simulink model "Computer"  (Simulink 8.1)
settings: Solver=ode45  StartTime=0.0  StopTime=21  RelTol=1e-3
libraries: Common_Library x33, commutil2 x5, Computer_Library x3, simulink_extras x3
settings Model: Creator=N  LastModifiedBy=uzivatel
settings DataIOCC: LimitDataPoints=off  SignalLoggingSaveFormat=Dataset
settings OptimizationCC: ExpressionDepthLimit=128
settings DebuggingCC: UnderspecifiedInitializationDetection=Simplified  MergeDetectMultiDrivingBlocksExec=error  SolverPrmCheckMsg=none  FcnCallInpInsideContextMsg=EnableAllAsError  FrameProcessingCompatibilityMsg=error  StateNameClashWarn=none
settings HardwareCC: ProdBitPerPointer=64  ProdLargestAtomicFloat=Float  ProdIntDivRoundTo=Zero  ProdEndianess=LittleEndian  ProdHWDeviceType=Intel->x86-64 (Windows64)
settings ModelReferenceCC: PropagateSignalLabelsOutOfModel=on
settings GRTTargetCC: CodeReplacementLibrary=None  CombineOutputUpdateFcns=on  CPPClassGenCompliant=on  GRTInterface=off

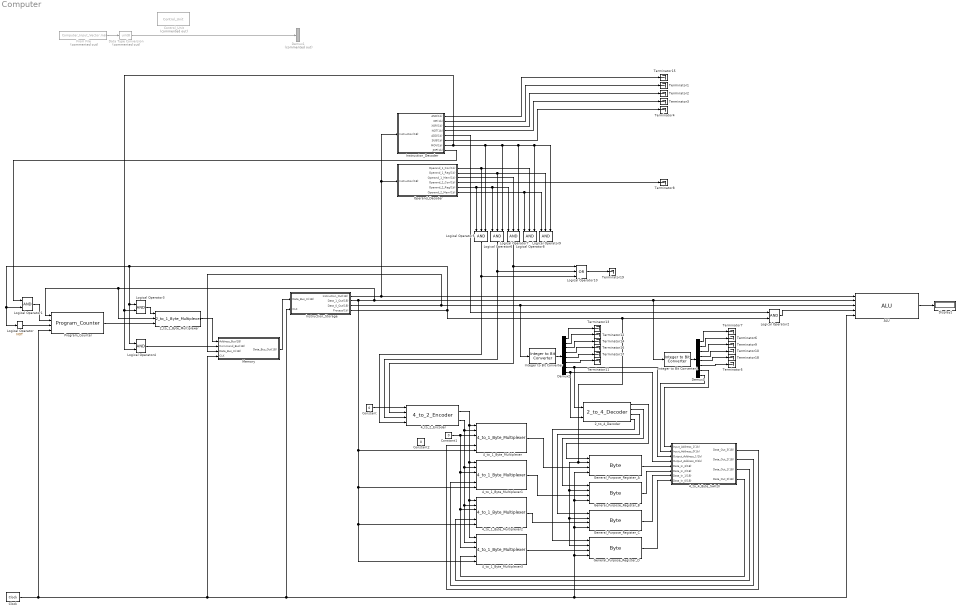
== system Computer ==
  2_to_1_Byte_Multiplexer : Common_Library/Multiplexers/2_to_1_Byte_Multiplexer
  2_to_4_Decoder : Common_Library/Decoders/2_to_4_Decoder
  4_to_1_Byte_Multiplexer{,1..3} (4 alike) : Common_Library/Multiplexers/4_to_1_Byte_Multiplexer
  4_to_2_Encoder : Common_Library/Encoders/4_to_2_Encoder
  4_to_4_Byte_Switch : Subsystem
  ALU : Computer_Library/ALU
  Clock : simulink_extras/Flip Flops/Clock  period=1
  Constant : Constant  Value=0  OutDataTypeStr=boolean
  Constant1 : Constant  Value=0  OutDataTypeStr=uint8
  Constant2 : Constant  Value=0  OutDataTypeStr=uint8
  Control_Unit : Computer_Library/Control_Unit  Commented=on
  Data Type Conversion : DataTypeConversion  Commented=on  OutDataTypeStr=uint8
  Demux1 : Demux  Commented=on  Outputs=2
  Demux2 : Demux  Outputs=8
  Demux3 : Demux  Outputs=8
  Display1 : Display
  From File : FromFile  Commented=on  FileName=Computer_Input_Vector.mat  OutDataTypeStr=double  SampleTime=1  ExtrapolationBeforeFirstDataPoint=Hold first value  ExtrapolationAfterLastDataPoint=Ground value
  General_Purpose_Register_A : Common_Library/Memory_Blocks/Byte
  General_Purpose_Register_B : Common_Library/Memory_Blocks/Byte
  General_Purpose_Register_C : Common_Library/Memory_Blocks/Byte
  General_Purpose_Register_D : Common_Library/Memory_Blocks/Byte
  Instruction_Decoder : Subsystem
  Instruction_Storage : Subsystem
  Integer to Bit Converter : commutil2/Integer to Bit Converter  nbits=8  signedInputValues=Unsigned  bitOrder=MSB first  outDtype=boolean
  Integer to Bit Converter1 : commutil2/Integer to Bit Converter  nbits=8  signedInputValues=Unsigned  bitOrder=MSB first  outDtype=boolean
  Logical Operator : Logic  Operator=NOT  IconShape=distinctive  AllPortsSameDT=off  OutDataTypeStr=boolean
  Logical Operator{1..4} (4 alike) : Logic  IconShape=distinctive  AllPortsSameDT=off  OutDataTypeStr=boolean
  Logical Operator10 : Logic  Operator=OR  Inputs=3  IconShape=distinctive  AllPortsSameDT=off  OutDataTypeStr=boolean
  Logical Operator{5..9} (5 alike) : Logic  Inputs=3  IconShape=distinctive  AllPortsSameDT=off  OutDataTypeStr=boolean
  Memory : Subsystem
  Operand_Decoder : Subsystem
  Program_Counter : Computer_Library/Program_Counter
  Terminator{1..19} (19 alike) : Terminator
  wires:
  Instruction_Storage/4(Process(1b)) -> Logical Operator4/1, Logical Operator3/1, Logical Operator/1, Logical Operator1/2, Logical Operator2/2, General_Purpose_Register_B/2, General_Purpose_Register_C/2, General_Purpose_Register_D/2, General_Purpose_Register_A/2
  Program_Counter/1 -> 2_to_1_Byte_Multiplexer/3
  Instruction_Storage/3(Data_0_Out(1B)) -> ALU/3, Integer to Bit Converter/1, Memory/3(Data_Bus_In(1B))
  Instruction_Decoder/8(JMP(1b)) -> Logical Operator1/1
  Instruction_Storage/2(Data_1_Out(1B)) -> 2_to_1_Byte_Multiplexer/2, Program_Counter/1, Integer to Bit Converter1/1, ALU/2, 4_to_1_Byte_Multiplexer3/6, 4_to_1_Byte_Multiplexer2/6, 4_to_1_Byte_Multiplexer1/6, 4_to_1_Byte_Multiplexer/6
  Memory/1(Data_Bus_Out(1B)) -> Instruction_Storage/1(Data_Bus_In(1B))
  Clock/1 -> Program_Counter/4, Memory/4(CLK), Instruction_Storage/2(CLK), ALU/5, General_Purpose_Register_A/4, General_Purpose_Register_B/4, General_Purpose_Register_C/4, General_Purpose_Register_D/4
  From File/1 -> Data Type Conversion/1
  Data Type Conversion/1 -> Demux1/1
  Instruction_Decoder/7(MOV(1b)) -> Logical Operator5/3, Logical Operator6/3, Logical Operator7/3, Logical Operator8/3, Logical Operator9/3, Logical Operator4/2, Logical Operator3/2
  Instruction_Storage/1(Instruction_Out(1B)) -> Operand_Decoder/1(Instruction(1B)), Instruction_Decoder/1(Instruction(1B)), ALU/1
  Logical Operator/1 -> Program_Counter/3
  Instruction_Decoder/5(ADD(1b)) -> Logical Operator2/1
  Logical Operator1/1 -> Program_Counter/2
  Logical Operator2/1 -> ALU/4
  2_to_1_Byte_Multiplexer/1 -> Memory/1(Address_Bus(1B))
  ALU/1 -> Display1/1
  Logical Operator3/1 -> 2_to_1_Byte_Multiplexer/1
  Logical Operator4/1 -> Memory/2(Command_Bus(1B))
  Instruction_Decoder/1(AND(1b)) -> Terminator15/1
  Instruction_Decoder/2(OR(1b)) -> Terminator1/1
  Instruction_Decoder/3(XOR(1b)) -> Terminator2/1
  Instruction_Decoder/4(NOT(1b)) -> Terminator3/1
  Instruction_Decoder/6(SUB(1b)) -> Terminator4/1
  Operand_Decoder/1(Operand_1_Con(1b)) -> Logical Operator8/2, Logical Operator5/2
  Operand_Decoder/2(Operand_1_Reg(1b)) -> Logical Operator6/2, Logical Operator9/2
  Operand_Decoder/3(Operand_1_Mem(1b)) -> Logical Operator7/2
  Operand_Decoder/4(Operand_2_Con(1b)) -> Terminator8/1
  Operand_Decoder/6(Operand_2_Mem(1b)) -> Logical Operator9/1, Logical Operator8/1
  2_to_4_Decoder/4 -> General_Purpose_Register_D/1
  2_to_4_Decoder/3 -> General_Purpose_Register_C/1
  2_to_4_Decoder/2 -> General_Purpose_Register_B/1
  2_to_4_Decoder/1 -> General_Purpose_Register_A/1
  Integer to Bit Converter/1 -> Demux2/1
  Demux2/8 -> 2_to_4_Decoder/2, 4_to_4_Byte_Switch/4(Output_Address_0(1b))
  Demux2/7 -> 2_to_4_Decoder/1, 4_to_4_Byte_Switch/3(Output_Address_1(1b))
  Demux2/1 -> Terminator13/1
  Demux2/2 -> Terminator12/1
  Demux2/3 -> Terminator14/1
  Demux2/4 -> Terminator16/1
  Demux2/5 -> Terminator17/1
  Demux2/6 -> Terminator11/1
  Operand_Decoder/5(Operand_2_Reg(1b)) -> Logical Operator7/1, Logical Operator6/1, Logical Operator5/1
  General_Purpose_Register_A/1 -> 4_to_4_Byte_Switch/5(Data_In_3(1B))
  General_Purpose_Register_B/1 -> 4_to_4_Byte_Switch/6(Data_In_2(1B))
  General_Purpose_Register_C/1 -> 4_to_4_Byte_Switch/7(Data_In_1(1B))
  General_Purpose_Register_D/1 -> 4_to_4_Byte_Switch/8(Data_In_0(1B))
  4_to_4_Byte_Switch/4(Data_Out_0(1B)) -> 4_to_1_Byte_Multiplexer3/5
  4_to_4_Byte_Switch/3(Data_Out_1(1B)) -> 4_to_1_Byte_Multiplexer2/5
  4_to_4_Byte_Switch/2(Data_Out_2(1B)) -> 4_to_1_Byte_Multiplexer1/5
  4_to_4_Byte_Switch/1(Data_Out_3(1B)) -> 4_to_1_Byte_Multiplexer/5
  Logical Operator5/1 -> Logical Operator10/3, 4_to_2_Encoder/4
  Logical Operator6/1 -> Logical Operator10/2, 4_to_2_Encoder/3
  Logical Operator7/1 -> Logical Operator10/1, 4_to_2_Encoder/2
  4_to_1_Byte_Multiplexer/1 -> General_Purpose_Register_A/3
  Constant/1 -> 4_to_2_Encoder/1
  4_to_1_Byte_Multiplexer1/1 -> General_Purpose_Register_B/3
  Constant1/1 -> 4_to_1_Byte_Multiplexer/3, 4_to_1_Byte_Multiplexer1/3, 4_to_1_Byte_Multiplexer2/3, 4_to_1_Byte_Multiplexer3/3
  4_to_1_Byte_Multiplexer2/1 -> General_Purpose_Register_C/3
  4_to_2_Encoder/1 -> 4_to_1_Byte_Multiplexer3/1, 4_to_1_Byte_Multiplexer2/1, 4_to_1_Byte_Multiplexer1/1, 4_to_1_Byte_Multiplexer/1
  4_to_2_Encoder/2 -> 4_to_1_Byte_Multiplexer3/2, 4_to_1_Byte_Multiplexer2/2, 4_to_1_Byte_Multiplexer1/2, 4_to_1_Byte_Multiplexer/2
  4_to_1_Byte_Multiplexer3/1 -> General_Purpose_Register_D/3
  Integer to Bit Converter1/1 -> Demux3/1
  Demux3/1 -> Terminator7/1
  Demux3/2 -> Terminator6/1
  Demux3/3 -> Terminator9/1
  Demux3/4 -> Terminator10/1
  Demux3/5 -> Terminator18/1
  Demux3/6 -> Terminator5/1
  Demux3/8 -> 4_to_4_Byte_Switch/2(Input_Address_0(1b))
  Demux3/7 -> 4_to_4_Byte_Switch/1(Input_Address_1(1b))
  Logical Operator10/1 -> Terminator19/1

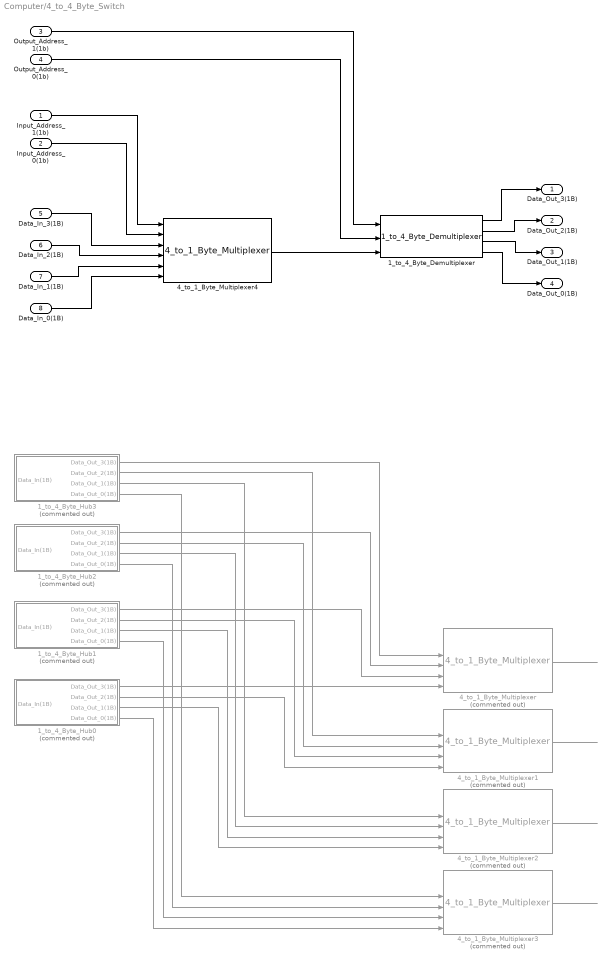
== system Computer/4_to_4_Byte_Switch ==
  Input_Address_1(1b) : Inport
  Input_Address_0(1b) : Inport  Port=2
  Output_Address_1(1b) : Inport  Port=3
  Output_Address_0(1b) : Inport  Port=4
  Data_In_3(1B) : Inport  Port=5
  Data_In_2(1B) : Inport  Port=6
  Data_In_1(1B) : Inport  Port=7
  Data_In_0(1B) : Inport  Port=8
  1_to_4_Byte_Demultiplexer : Common_Library/Demultiplexers/1_to_4_Byte_Demultiplexer
  1_to_4_Byte_Hub0 : Subsystem  Commented=on
  1_to_4_Byte_Hub1 : Subsystem  Commented=on
  1_to_4_Byte_Hub2 : Subsystem  Commented=on
  1_to_4_Byte_Hub3 : Subsystem  Commented=on
  4_to_1_Byte_Multiplexer{,1..3} (4 alike) : Common_Library/Multiplexers/4_to_1_Byte_Multiplexer  Commented=on
  4_to_1_Byte_Multiplexer4 : Common_Library/Multiplexers/4_to_1_Byte_Multiplexer
  Data_Out_3(1B) : Outport
  Data_Out_2(1B) : Outport  Port=2
  Data_Out_1(1B) : Outport  Port=3
  Data_Out_0(1B) : Outport  Port=4
  wires:
  4_to_1_Byte_Multiplexer/1 -> ?
  1_to_4_Byte_Hub3/1(Data_Out_3(1B)) -> 4_to_1_Byte_Multiplexer/3
  1_to_4_Byte_Hub2/1(Data_Out_3(1B)) -> 4_to_1_Byte_Multiplexer/4
  1_to_4_Byte_Hub1/1(Data_Out_3(1B)) -> 4_to_1_Byte_Multiplexer/5
  1_to_4_Byte_Hub0/1(Data_Out_3(1B)) -> 4_to_1_Byte_Multiplexer/6
  ? -> 1_to_4_Byte_Hub3/1(Data_In(1B))
  ? -> 1_to_4_Byte_Hub2/1(Data_In(1B))
  ? -> 1_to_4_Byte_Hub1/1(Data_In(1B))
  ? -> 1_to_4_Byte_Hub0/1(Data_In(1B))
  4_to_1_Byte_Multiplexer1/1 -> ?
  4_to_1_Byte_Multiplexer2/1 -> ?
  4_to_1_Byte_Multiplexer3/1 -> ?
  1_to_4_Byte_Hub3/2(Data_Out_2(1B)) -> 4_to_1_Byte_Multiplexer1/3
  1_to_4_Byte_Hub2/2(Data_Out_2(1B)) -> 4_to_1_Byte_Multiplexer1/4
  1_to_4_Byte_Hub1/2(Data_Out_2(1B)) -> 4_to_1_Byte_Multiplexer1/5
  1_to_4_Byte_Hub0/2(Data_Out_2(1B)) -> 4_to_1_Byte_Multiplexer1/6
  1_to_4_Byte_Hub3/3(Data_Out_1(1B)) -> 4_to_1_Byte_Multiplexer2/3
  1_to_4_Byte_Hub2/3(Data_Out_1(1B)) -> 4_to_1_Byte_Multiplexer2/4
  1_to_4_Byte_Hub1/3(Data_Out_1(1B)) -> 4_to_1_Byte_Multiplexer2/5
  1_to_4_Byte_Hub0/3(Data_Out_1(1B)) -> 4_to_1_Byte_Multiplexer2/6
  1_to_4_Byte_Hub3/4(Data_Out_0(1B)) -> 4_to_1_Byte_Multiplexer3/3
  1_to_4_Byte_Hub2/4(Data_Out_0(1B)) -> 4_to_1_Byte_Multiplexer3/4
  1_to_4_Byte_Hub1/4(Data_Out_0(1B)) -> 4_to_1_Byte_Multiplexer3/5
  1_to_4_Byte_Hub0/4(Data_Out_0(1B)) -> 4_to_1_Byte_Multiplexer3/6
  ? -> 4_to_1_Byte_Multiplexer/2, 4_to_1_Byte_Multiplexer1/2, 4_to_1_Byte_Multiplexer2/2, 4_to_1_Byte_Multiplexer3/2
  ? -> 4_to_1_Byte_Multiplexer/1, 4_to_1_Byte_Multiplexer1/1, 4_to_1_Byte_Multiplexer2/1, 4_to_1_Byte_Multiplexer3/1
  4_to_1_Byte_Multiplexer4/1 -> 1_to_4_Byte_Demultiplexer/3
  1_to_4_Byte_Demultiplexer/1 -> Data_Out_3(1B)/1
  1_to_4_Byte_Demultiplexer/2 -> Data_Out_2(1B)/1
  1_to_4_Byte_Demultiplexer/3 -> Data_Out_1(1B)/1
  1_to_4_Byte_Demultiplexer/4 -> Data_Out_0(1B)/1
  Data_In_0(1B)/1 -> 4_to_1_Byte_Multiplexer4/6
  Data_In_1(1B)/1 -> 4_to_1_Byte_Multiplexer4/5
  Data_In_2(1B)/1 -> 4_to_1_Byte_Multiplexer4/4
  Data_In_3(1B)/1 -> 4_to_1_Byte_Multiplexer4/3
  Input_Address_0(1b)/1 -> 4_to_1_Byte_Multiplexer4/2
  Input_Address_1(1b)/1 -> 4_to_1_Byte_Multiplexer4/1
  Output_Address_0(1b)/1 -> 1_to_4_Byte_Demultiplexer/2
  Output_Address_1(1b)/1 -> 1_to_4_Byte_Demultiplexer/1

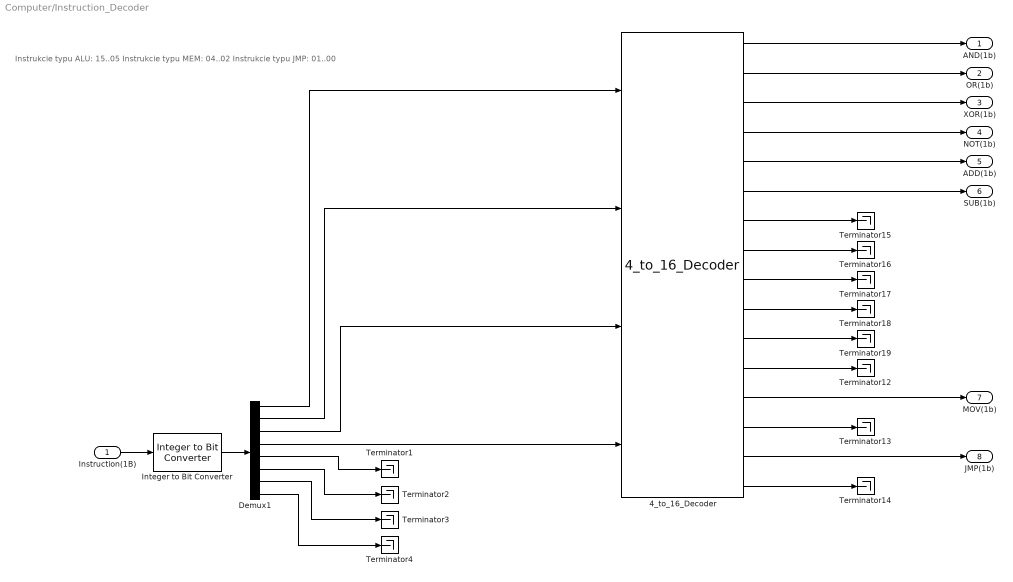
== system Computer/Instruction_Decoder ==
  note: Instrukcie typu ALU: 15..05
      | Instrukcie typu MEM: 04..02
      | Instrukcie typu JMP: 01..00
  Instruction(1B) : Inport
  4_to_16_Decoder : Common_Library/Decoders/4_to_16_Decoder
  Demux1 : Demux  Outputs=8
  Integer to Bit Converter : commutil2/Integer to Bit Converter  nbits=8  signedInputValues=Unsigned  bitOrder=MSB first  outDtype=boolean
  Terminator{1..4,12..19} (12 alike) : Terminator
  AND(1b) : Outport
  OR(1b) : Outport  Port=2
  XOR(1b) : Outport  Port=3
  NOT(1b) : Outport  Port=4
  ADD(1b) : Outport  Port=5
  SUB(1b) : Outport  Port=6
  MOV(1b) : Outport  Port=7
  JMP(1b) : Outport  Port=8
  wires:
  4_to_16_Decoder/5 -> ADD(1b)/1
  Instruction(1B)/1 -> Integer to Bit Converter/1
  Demux1/5 -> Terminator1/1
  Demux1/1 -> 4_to_16_Decoder/1
  Demux1/2 -> 4_to_16_Decoder/2
  Demux1/3 -> 4_to_16_Decoder/3
  Demux1/4 -> 4_to_16_Decoder/4
  Integer to Bit Converter/1 -> Demux1/1
  4_to_16_Decoder/15 -> JMP(1b)/1
  4_to_16_Decoder/13 -> MOV(1b)/1
  4_to_16_Decoder/1 -> AND(1b)/1
  4_to_16_Decoder/2 -> OR(1b)/1
  4_to_16_Decoder/3 -> XOR(1b)/1
  4_to_16_Decoder/4 -> NOT(1b)/1
  4_to_16_Decoder/7 -> Terminator15/1
  4_to_16_Decoder/8 -> Terminator16/1
  4_to_16_Decoder/9 -> Terminator17/1
  4_to_16_Decoder/10 -> Terminator18/1
  4_to_16_Decoder/11 -> Terminator19/1
  4_to_16_Decoder/12 -> Terminator12/1
  4_to_16_Decoder/14 -> Terminator13/1
  4_to_16_Decoder/16 -> Terminator14/1
  4_to_16_Decoder/6 -> SUB(1b)/1
  Demux1/6 -> Terminator2/1
  Demux1/7 -> Terminator3/1
  Demux1/8 -> Terminator4/1

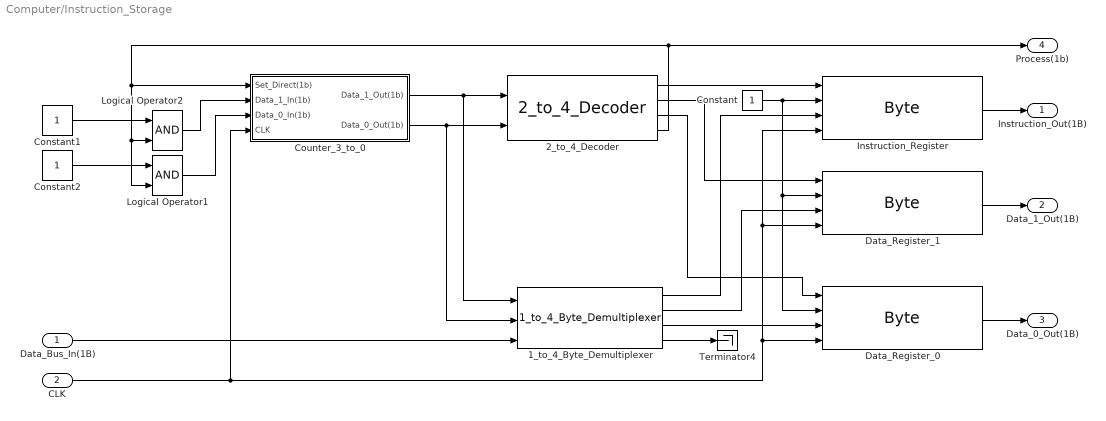
== system Computer/Instruction_Storage ==
  Data_Bus_In(1B) : Inport
  CLK : Inport  Port=2
  1_to_4_Byte_Demultiplexer : Common_Library/Demultiplexers/1_to_4_Byte_Demultiplexer
  2_to_4_Decoder : Common_Library/Decoders/2_to_4_Decoder
  Constant : Constant  OutDataTypeStr=boolean
  Constant1 : Constant  OutDataTypeStr=uint8
  Constant2 : Constant  OutDataTypeStr=uint8
  Counter_3_to_0 : Subsystem
  Data_Register_0 : Common_Library/Memory_Blocks/Byte
  Data_Register_1 : Common_Library/Memory_Blocks/Byte
  Instruction_Register : Common_Library/Memory_Blocks/Byte
  Logical Operator1 : Logic  IconShape=distinctive  AllPortsSameDT=off  OutDataTypeStr=boolean
  Logical Operator2 : Logic  IconShape=distinctive  AllPortsSameDT=off  OutDataTypeStr=boolean
  Terminator4 : Terminator
  Instruction_Out(1B) : Outport
  Data_1_Out(1B) : Outport  Port=2
  Data_0_Out(1B) : Outport  Port=3
  Process(1b) : Outport  Port=4
  wires:
  Logical Operator1/1 -> Counter_3_to_0/3(Data_0_In(1b))
  Logical Operator2/1 -> Counter_3_to_0/2(Data_1_In(1b))
  2_to_4_Decoder/4 -> Logical Operator1/2, Logical Operator2/2, Counter_3_to_0/1(Set_Direct(1b)), Process(1b)/1
  Data_Register_0/1 -> Data_0_Out(1B)/1
  Data_Register_1/1 -> Data_1_Out(1B)/1
  Instruction_Register/1 -> Instruction_Out(1B)/1
  1_to_4_Byte_Demultiplexer/4 -> Terminator4/1
  Counter_3_to_0/1(Data_1_Out(1b)) -> 2_to_4_Decoder/1, 1_to_4_Byte_Demultiplexer/1
  Counter_3_to_0/2(Data_0_Out(1b)) -> 2_to_4_Decoder/2, 1_to_4_Byte_Demultiplexer/2
  Data_Bus_In(1B)/1 -> 1_to_4_Byte_Demultiplexer/3
  Constant/1 -> Instruction_Register/2, Data_Register_0/2, Data_Register_1/2
  1_to_4_Byte_Demultiplexer/3 -> Data_Register_0/3
  CLK/1 -> Data_Register_1/4, Instruction_Register/4, Data_Register_0/4, Counter_3_to_0/4(CLK)
  Constant1/1 -> Logical Operator2/1
  Constant2/1 -> Logical Operator1/1
  1_to_4_Byte_Demultiplexer/2 -> Data_Register_1/3
  1_to_4_Byte_Demultiplexer/1 -> Instruction_Register/3
  2_to_4_Decoder/1 -> Instruction_Register/1
  2_to_4_Decoder/2 -> Data_Register_1/1
  2_to_4_Decoder/3 -> Data_Register_0/1

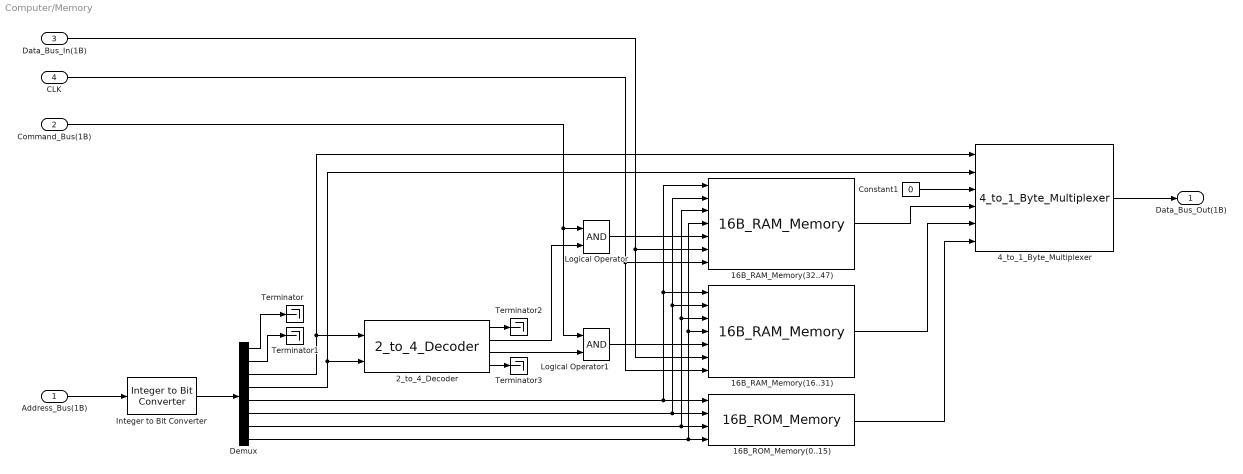
== system Computer/Memory ==
  Address_Bus(1B) : Inport
  Command_Bus(1B) : Inport  Port=2
  Data_Bus_In(1B) : Inport  Port=3
  CLK : Inport  Port=4
  16B_RAM_Memory(16..31) : Common_Library/Memory_Blocks/16B_RAM_Memory
  16B_RAM_Memory(32..47) : Common_Library/Memory_Blocks/16B_RAM_Memory
  16B_ROM_Memory(0..15) : Common_Library/Memory_Blocks/16B_ROM_Memory
  2_to_4_Decoder : Common_Library/Decoders/2_to_4_Decoder
  4_to_1_Byte_Multiplexer : Common_Library/Multiplexers/4_to_1_Byte_Multiplexer
  Constant1 : Constant  Value=0  OutDataTypeStr=uint8
  Demux : Demux  Outputs=8
  Integer to Bit Converter : commutil2/Integer to Bit Converter  nbits=8  signedInputValues=Unsigned  bitOrder=MSB first  outDtype=boolean
  Logical Operator : Logic  IconShape=distinctive  AllPortsSameDT=off  OutDataTypeStr=boolean
  Logical Operator1 : Logic  IconShape=distinctive  AllPortsSameDT=off  OutDataTypeStr=boolean
  Terminator{,1..3} (4 alike) : Terminator
  Data_Bus_Out(1B) : Outport
  wires:
  4_to_1_Byte_Multiplexer/1 -> Data_Bus_Out(1B)/1
  16B_ROM_Memory(0..15)/1 -> 4_to_1_Byte_Multiplexer/6
  16B_RAM_Memory(16..31)/1 -> 4_to_1_Byte_Multiplexer/5
  Demux/8 -> 16B_RAM_Memory(16..31)/4, 16B_RAM_Memory(32..47)/4, 16B_ROM_Memory(0..15)/4
  Demux/7 -> 16B_RAM_Memory(32..47)/3, 16B_RAM_Memory(16..31)/3, 16B_ROM_Memory(0..15)/3
  Demux/6 -> 16B_RAM_Memory(32..47)/2, 16B_RAM_Memory(16..31)/2, 16B_ROM_Memory(0..15)/2
  Demux/5 -> 16B_RAM_Memory(32..47)/1, 16B_RAM_Memory(16..31)/1, 16B_ROM_Memory(0..15)/1
  Demux/4 -> 2_to_4_Decoder/2, 4_to_1_Byte_Multiplexer/2
  Demux/2 -> Terminator1/1
  Demux/1 -> Terminator/1
  Demux/3 -> 4_to_1_Byte_Multiplexer/1, 2_to_4_Decoder/1
  16B_RAM_Memory(32..47)/1 -> 4_to_1_Byte_Multiplexer/4
  Data_Bus_In(1B)/1 -> 16B_RAM_Memory(32..47)/6, 16B_RAM_Memory(16..31)/6
  Integer to Bit Converter/1 -> Demux/1
  CLK/1 -> 16B_RAM_Memory(16..31)/7, 16B_RAM_Memory(32..47)/7
  2_to_4_Decoder/3 -> Logical Operator1/2
  2_to_4_Decoder/2 -> Logical Operator/2
  2_to_4_Decoder/4 -> Terminator3/1
  2_to_4_Decoder/1 -> Terminator2/1
  Logical Operator/1 -> 16B_RAM_Memory(32..47)/5
  Logical Operator1/1 -> 16B_RAM_Memory(16..31)/5
  Command_Bus(1B)/1 -> Logical Operator/1, Logical Operator1/1
  Address_Bus(1B)/1 -> Integer to Bit Converter/1
  Constant1/1 -> 4_to_1_Byte_Multiplexer/3

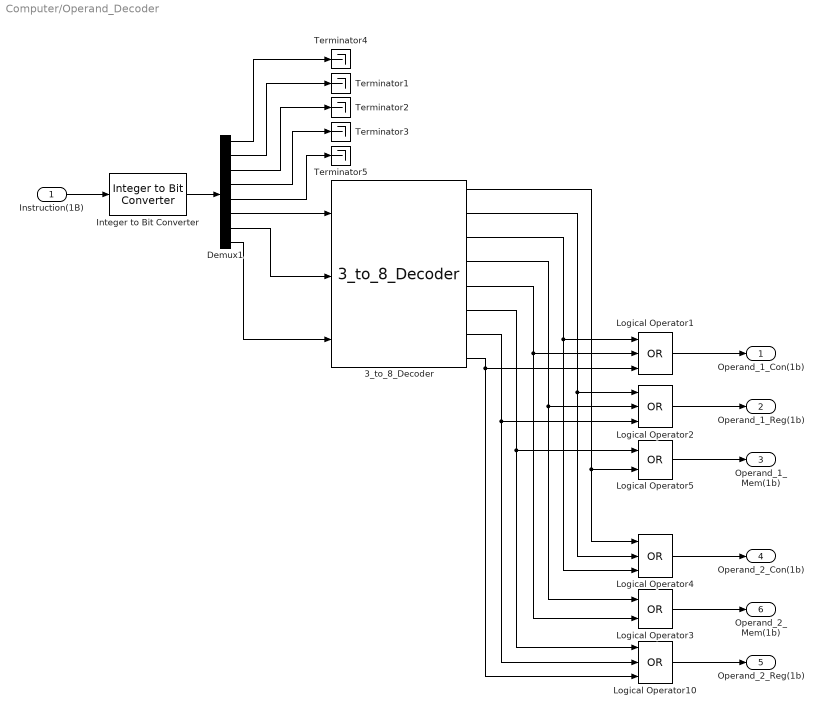
== system Computer/Operand_Decoder ==
  Instruction(1B) : Inport
  3_to_8_Decoder : Common_Library/Decoders/3_to_8_Decoder
  Demux1 : Demux  Outputs=8
  Integer to Bit Converter : commutil2/Integer to Bit Converter  nbits=8  signedInputValues=Unsigned  bitOrder=MSB first  outDtype=boolean
  Logical Operator{1..2,4,10} (4 alike) : Logic  Operator=OR  Inputs=3  IconShape=distinctive  AllPortsSameDT=off  OutDataTypeStr=boolean
  Logical Operator3 : Logic  Operator=OR  IconShape=distinctive  AllPortsSameDT=off  OutDataTypeStr=boolean
  Logical Operator5 : Logic  Operator=OR  IconShape=distinctive  AllPortsSameDT=off  OutDataTypeStr=boolean
  Terminator{1..5} (5 alike) : Terminator
  Operand_1_Con(1b) : Outport
  Operand_1_Reg(1b) : Outport  Port=2
  Operand_1_Mem(1b) : Outport  Port=3
  Operand_2_Con(1b) : Outport  Port=4
  Operand_2_Reg(1b) : Outport  Port=5
  Operand_2_Mem(1b) : Outport  Port=6
  wires:
  Demux1/8 -> 3_to_8_Decoder/3
  Demux1/7 -> 3_to_8_Decoder/2
  Demux1/6 -> 3_to_8_Decoder/1
  Logical Operator4/1 -> Operand_2_Con(1b)/1
  3_to_8_Decoder/8 -> Logical Operator10/3, Logical Operator1/3
  3_to_8_Decoder/2 -> Logical Operator4/2, Logical Operator2/1
  3_to_8_Decoder/7 -> Logical Operator10/2, Logical Operator2/3
  Logical Operator2/1 -> Operand_1_Reg(1b)/1
  3_to_8_Decoder/5 -> Logical Operator3/2, Logical Operator1/2
  Logical Operator10/1 -> Operand_2_Reg(1b)/1
  3_to_8_Decoder/4 -> Logical Operator3/1, Logical Operator2/2
  3_to_8_Decoder/6 -> Logical Operator10/1, Logical Operator5/1
  Logical Operator3/1 -> Operand_2_Mem(1b)/1
  Logical Operator1/1 -> Operand_1_Con(1b)/1
  3_to_8_Decoder/1 -> Logical Operator4/1, Logical Operator5/2
  3_to_8_Decoder/3 -> Logical Operator4/3, Logical Operator1/1
  Logical Operator5/1 -> Operand_1_Mem(1b)/1
  Instruction(1B)/1 -> Integer to Bit Converter/1
  Integer to Bit Converter/1 -> Demux1/1
  Demux1/1 -> Terminator4/1
  Demux1/2 -> Terminator1/1
  Demux1/3 -> Terminator2/1
  Demux1/4 -> Terminator3/1
  Demux1/5 -> Terminator5/1

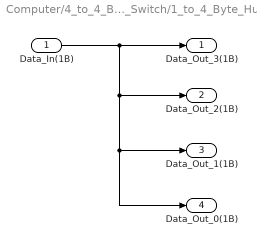
== system Computer/4_to_4_Byte_Switch/1_to_4_Byte_Hub0 ==
  Data_In(1B) : Inport
  Data_Out_3(1B) : Outport
  Data_Out_2(1B) : Outport  Port=2
  Data_Out_1(1B) : Outport  Port=3
  Data_Out_0(1B) : Outport  Port=4
  wires:
  Data_In(1B)/1 -> Data_Out_2(1B)/1, Data_Out_1(1B)/1, Data_Out_0(1B)/1, Data_Out_3(1B)/1

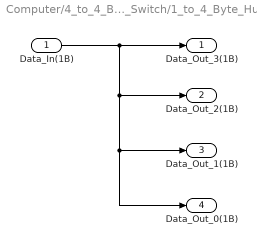
== system Computer/4_to_4_Byte_Switch/1_to_4_Byte_Hub1 ==
  Data_In(1B) : Inport
  Data_Out_3(1B) : Outport
  Data_Out_2(1B) : Outport  Port=2
  Data_Out_1(1B) : Outport  Port=3
  Data_Out_0(1B) : Outport  Port=4
  wires:
  Data_In(1B)/1 -> Data_Out_2(1B)/1, Data_Out_1(1B)/1, Data_Out_0(1B)/1, Data_Out_3(1B)/1

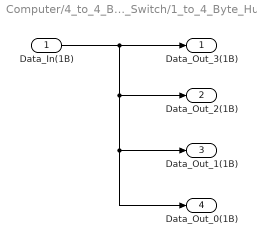
== system Computer/4_to_4_Byte_Switch/1_to_4_Byte_Hub2 ==
  Data_In(1B) : Inport
  Data_Out_3(1B) : Outport
  Data_Out_2(1B) : Outport  Port=2
  Data_Out_1(1B) : Outport  Port=3
  Data_Out_0(1B) : Outport  Port=4
  wires:
  Data_In(1B)/1 -> Data_Out_2(1B)/1, Data_Out_1(1B)/1, Data_Out_0(1B)/1, Data_Out_3(1B)/1

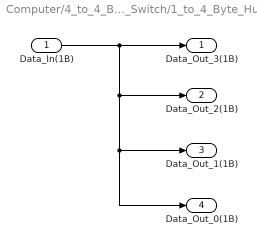
== system Computer/4_to_4_Byte_Switch/1_to_4_Byte_Hub3 ==
  Data_In(1B) : Inport
  Data_Out_3(1B) : Outport
  Data_Out_2(1B) : Outport  Port=2
  Data_Out_1(1B) : Outport  Port=3
  Data_Out_0(1B) : Outport  Port=4
  wires:
  Data_In(1B)/1 -> Data_Out_2(1B)/1, Data_Out_1(1B)/1, Data_Out_0(1B)/1, Data_Out_3(1B)/1

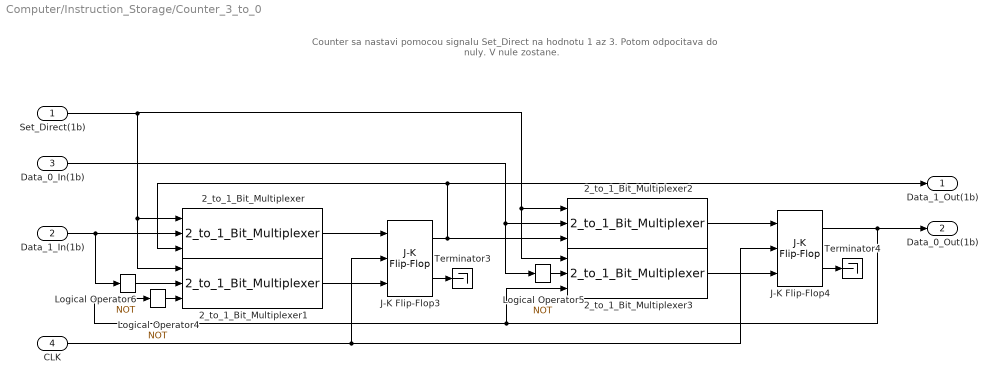
== system Computer/Instruction_Storage/Counter_3_to_0 ==
  note: Counter sa nastavi pomocou signalu Set_Direct na hodnotu 1 az 3.
      | Potom odpocitava do nuly. V nule zostane.
  Set_Direct(1b) : Inport
  Data_1_In(1b) : Inport  Port=2
  Data_0_In(1b) : Inport  Port=3
  CLK : Inport  Port=4
  2_to_1_Bit_Multiplexer{,1..3} (4 alike) : Common_Library/Multiplexers/2_to_1_Bit_Multiplexer
  J-K Flip-Flop3 : simulink_extras/Flip Flops/J-K Flip-Flop  initial_condition=0
  J-K Flip-Flop4 : simulink_extras/Flip Flops/J-K Flip-Flop  initial_condition=0
  Logical Operator4 : Logic  Operator=NOT  IconShape=distinctive  AllPortsSameDT=off  OutDataTypeStr=boolean
  Logical Operator5 : Logic  Operator=NOT  IconShape=distinctive  AllPortsSameDT=off  OutDataTypeStr=boolean
  Logical Operator6 : Logic  Operator=NOT  IconShape=distinctive  AllPortsSameDT=off  OutDataTypeStr=boolean
  Terminator3 : Terminator
  Terminator4 : Terminator
  Data_1_Out(1b) : Outport
  Data_0_Out(1b) : Outport  Port=2
  wires:
  2_to_1_Bit_Multiplexer3/1 -> J-K Flip-Flop4/3
  2_to_1_Bit_Multiplexer2/1 -> J-K Flip-Flop4/1
  Logical Operator5/1 -> 2_to_1_Bit_Multiplexer3/2
  Data_0_In(1b)/1 -> Logical Operator5/1, 2_to_1_Bit_Multiplexer2/2
  Set_Direct(1b)/1 -> 2_to_1_Bit_Multiplexer2/1, 2_to_1_Bit_Multiplexer3/1, 2_to_1_Bit_Multiplexer/1, 2_to_1_Bit_Multiplexer1/1
  Data_1_In(1b)/1 -> 2_to_1_Bit_Multiplexer/2, Logical Operator6/1
  2_to_1_Bit_Multiplexer1/1 -> J-K Flip-Flop3/3
  2_to_1_Bit_Multiplexer/1 -> J-K Flip-Flop3/1
  Logical Operator6/1 -> 2_to_1_Bit_Multiplexer1/2
  J-K Flip-Flop3/2 -> Terminator3/1
  CLK/1 -> J-K Flip-Flop3/2, J-K Flip-Flop4/2
  J-K Flip-Flop4/1 -> Logical Operator4/1, 2_to_1_Bit_Multiplexer3/3, Data_0_Out(1b)/1
  Logical Operator4/1 -> 2_to_1_Bit_Multiplexer1/3
  J-K Flip-Flop3/1 -> 2_to_1_Bit_Multiplexer2/3, 2_to_1_Bit_Multiplexer/3, Data_1_Out(1b)/1
  J-K Flip-Flop4/2 -> Terminator4/1
